simulink subsystem "CMS"  (R2024b)
settings: Solver=VariableStepAuto  StartTime=0.0  StopTime=10.0  RelTol=1e-3
undefined symbols (not defined in the file): Ts
settings Model: Creator=Kyle  LastModifiedBy=CD8435

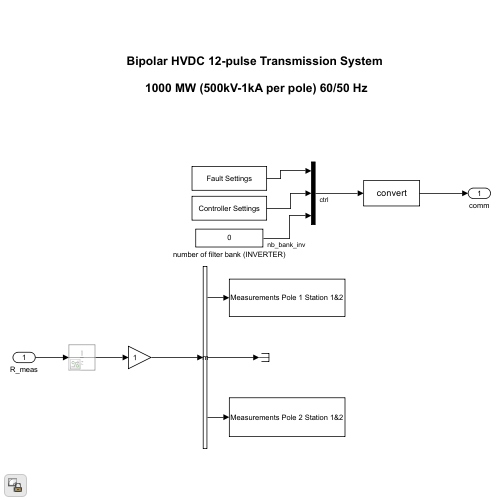
[thumbnail: Simulink's stored preview of the top-level diagram]
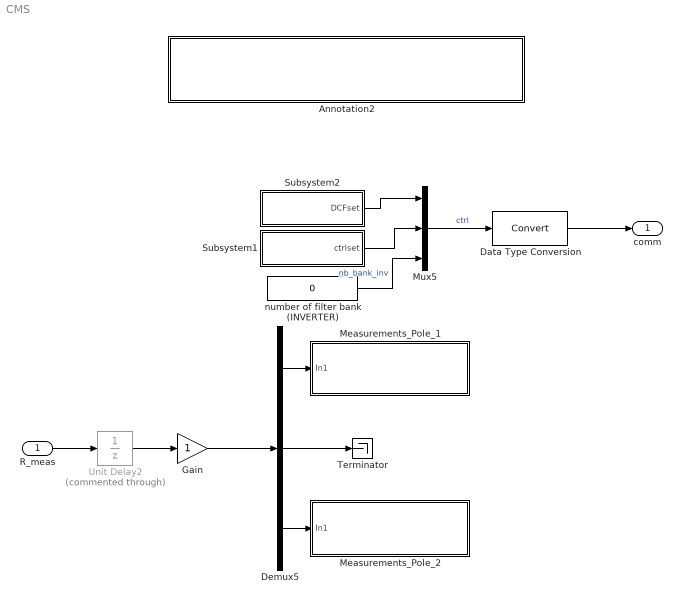
== system CMS ==
  R_meas : Inport
  Annotation2 : Subsystem  mask(Annotation){desc=|, maj=off, HZ=center, color=[0.9 0.9 0.9]}
      mask desc=|
      | Bipolar HVDC 12-pulse Transmission System
      | \n 1000 MW (500kV-1kA per pole) 60/50 Hz
      mask prompts: desc "Description (use \n for line return) :"; maj "Capital letters ?"; HZ "Horizontal Alignment"; color "Color [R G B] :"
      mask help: Annotation
      mask init:
      | if maj == 1 desc =upper(desc); end;
      | if strcmp(HZ, 'left') x = 0.05; end;
      | if strcmp(HZ, 'right') x = 0.95; end;
      | if strcmp(HZ, 'center') x = 0.50; end;
      mask TypeOptions HZ: left | right | center
      mask Display:
      | text(x, 0.50, desc, ...
      | 'horizontalAlignment', HZ, ...
      | 'verticalAlignment', 'middle') ;
  Data Type Conversion : DataTypeConversion  SaturateOnIntegerOverflow=off  RndMeth=Floor
  Demux5 : Demux  Outputs=[56 1 56]
      settings: DisplayOption=none
  Gain : Gain
  Measurements_Pole_1 : Subsystem
      mask Display: disp('Measurements Pole 1 Station 1&2')
  Measurements_Pole_2 : Subsystem
      mask Display: disp('Measurements Pole 2 Station 1&2')
  Mux5 : Mux  Inputs=3
  Subsystem1 : Subsystem
      mask Display: disp('Controller Settings')
  Subsystem2 : Subsystem
      mask Display: disp('Fault Settings')
  Terminator : Terminator
  Unit Delay2 : UnitDelay  Commented=through  SampleTime=Ts  HasFrameUpgradeWarning=on
  number of filter bank (INVERTER) : Constant  Value=0
  comm : Outport
  wires:
  Subsystem1/1(ctrlset) -> Mux5/2
  Subsystem2/1(DCFset) -> Mux5/1
  Mux5/1 -> Data Type Conversion/1  "ctrl"
  R_meas/1 -> Unit Delay2/1
  Demux5/1 -> Measurements_Pole_1/1(In1)
  Demux5/3 -> Measurements_Pole_2/1(In1)
  Demux5/2 -> Terminator/1
  Unit Delay2/1 -> Gain/1
  Gain/1 -> Demux5/1
  Data Type Conversion/1 -> comm/1
  number of filter bank (INVERTER)/1 -> Mux5/3  "nb_bank_inv"

== system CMS/Annotation2 ==
  note: Used only to display simulation parameters
  note: Text :
      | - justife a gauche
      | - Tahoma 10 Bold

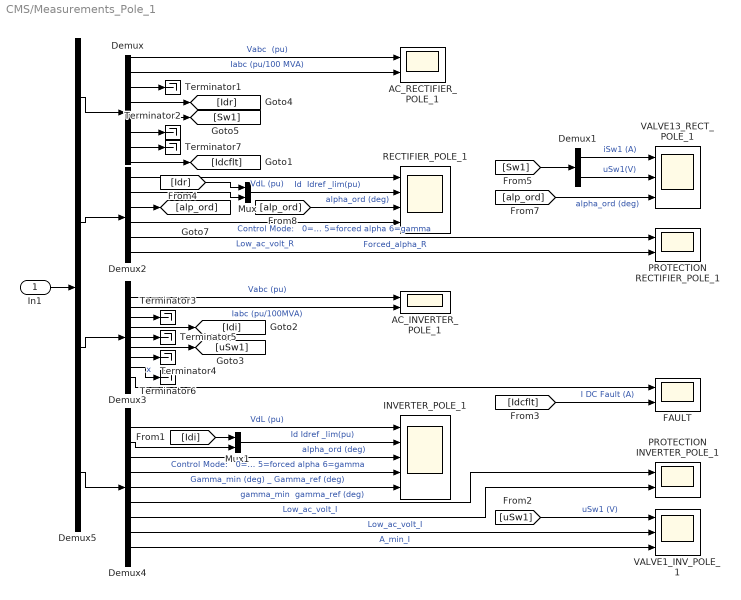
== system CMS/Measurements_Pole_1 ==
  In1 : Inport
  AC_INVERTER_POLE_1 : Scope  NumInputPorts=2
  AC_RECTIFIER_POLE_1 : Scope  NumInputPorts=2
  Demux : Demux  Outputs=[3 3 1 1 2 2 1 1]
  Demux1 : Demux  Outputs=[1 1]
      settings: DisplayOption=none
  Demux2 : Demux  Outputs=6
  Demux3 : Demux  Outputs="[3 3 1 1 12 1  1 1 1]"
  Demux4 : Demux  Outputs=[ 2 1 1 1 2 1 1 2 1]
  Demux5 : Demux  Outputs=[14 6 24 12]
      settings: DisplayOption=none
  FAULT : Scope  NumInputPorts=2
  INVERTER_POLE_1 : Scope  NumInputPorts=5
  Mux : Mux  Inputs=2
  Mux1 : Mux  Inputs=2
  PROTECTION INVERTER_POLE_1 : Scope  NumInputPorts=2
  PROTECTION RECTIFIER_POLE_1 : Scope  NumInputPorts=2
  RECTIFIER_POLE_1 : Scope  NumInputPorts=4
  Terminator{1..7} (7 alike) : Terminator
  VALVE13_RECT_POLE_1 : Scope  NumInputPorts=3
  VALVE1_INV_POLE_1 : Scope  NumInputPorts=3
  wires:
  In1/1 -> Demux5/1
  Demux/7 -> Terminator7/1
  Demux/8 -> [Idcflt]
  Demux3/8 -> Terminator6/1  "x"
  Demux3/9 -> FAULT/1
  [alp_ord] -> RECTIFIER_POLE_1/3  "alpha_ord (deg)"
  Demux2/3 -> [alp_ord]
  [alp_ord] -> VALVE13_RECT_POLE_1/3  "alpha_ord (deg)"
  [Sw1] -> Demux1/1
  [Idr] -> Mux/1
  [uSw1] -> VALVE1_INV_POLE_1/1  "uSw1 (V)"
  [Idi] -> Mux1/1
  [Idcflt] -> FAULT/2  "I DC Fault (A)"
  Demux3/7 -> Terminator4/1
  Demux5/4 -> Demux4/1
  Demux5/3 -> Demux3/1
  Demux5/2 -> Demux2/1
  Demux5/1 -> Demux/1
  Demux4/9 -> VALVE1_INV_POLE_1/3  "A_min_I"
  Demux4/7 -> PROTECTION INVERTER_POLE_1/2  "Low_ac_volt_I"
  Demux4/6 -> PROTECTION INVERTER_POLE_1/1  "gamma_min  gamma_ref (deg)"
  Demux3/5 -> Terminator5/1
  Demux3/3 -> Terminator3/1
  Demux3/6 -> [uSw1]
  Demux3/4 -> [Idi]
  Demux/6 -> Terminator2/1
  Demux/3 -> Terminator1/1
  Demux2/6 -> PROTECTION RECTIFIER_POLE_1/2  "Forced_alpha_R"
  Demux/4 -> [Idr]
  Demux/5 -> [Sw1]
  Demux4/8 -> VALVE1_INV_POLE_1/2  "Low_ac_volt_I"
  Demux1/2 -> VALVE13_RECT_POLE_1/2  "uSw1(V)"
  Demux1/1 -> VALVE13_RECT_POLE_1/1  "iSw1 (A)"
  Demux4/5 -> INVERTER_POLE_1/5  "Gamma_min (deg) _ Gamma_ref (deg)"
  Demux4/1 -> INVERTER_POLE_1/1  "VdL (pu)"
  Demux4/4 -> INVERTER_POLE_1/4  "Control Mode:   0=blked  1=curr 2=volt 3=alpha min  4=alpha max 5=forced alpha 6=gamma"
  Mux1/1 -> INVERTER_POLE_1/2  "Id Idref _lim(pu)"
  Demux4/2 -> Mux1/2
  Demux2/2 -> Mux/2
  Mux/1 -> RECTIFIER_POLE_1/2  "Id  Idref _lim(pu)"
  Demux2/5 -> PROTECTION RECTIFIER_POLE_1/1  "Low_ac_volt_R"
  Demux/1 -> AC_RECTIFIER_POLE_1/1  "Vabc  (pu)"
  Demux/2 -> AC_RECTIFIER_POLE_1/2  "Iabc (pu/100 MVA)"
  Demux2/1 -> RECTIFIER_POLE_1/1  "VdL (pu)"
  Demux3/1 -> AC_INVERTER_POLE_1/1  "Vabc (pu)"
  Demux3/2 -> AC_INVERTER_POLE_1/2  "Iabc (pu/100MVA)"
  Demux4/3 -> INVERTER_POLE_1/3  "alpha_ord (deg)"
  Demux2/4 -> RECTIFIER_POLE_1/4  "Control Mode:   0=blked  1=curr 2=volt 3=alpha min  4=alpha max 5=forced alpha 6=gamma"

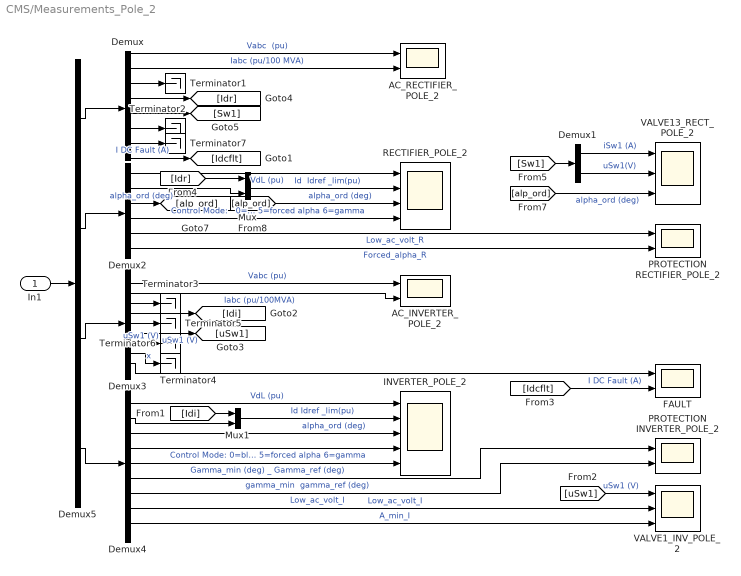
== system CMS/Measurements_Pole_2 ==
  In1 : Inport
  AC_INVERTER_POLE_2 : Scope  NumInputPorts=2
  AC_RECTIFIER_POLE_2 : Scope  NumInputPorts=2
  Demux : Demux  Outputs=[3 3 1 1 2 2 1 1]
  Demux1 : Demux  Outputs=[1 1]
      settings: DisplayOption=none
  Demux2 : Demux  Outputs=6
  Demux3 : Demux  Outputs="[3 3 1 1 12 1  1 1 1]"
  Demux4 : Demux  Outputs=[ 2 1 1 1 2 1 1 2 1]
  Demux5 : Demux  Outputs=[14 6 24 12]
      settings: DisplayOption=none
  FAULT : Scope  NumInputPorts=2
  INVERTER_POLE_2 : Scope  NumInputPorts=5
  Mux : Mux  Inputs=2
  Mux1 : Mux  Inputs=2
  PROTECTION INVERTER_POLE_2 : Scope  NumInputPorts=2
  PROTECTION RECTIFIER_POLE_2 : Scope  NumInputPorts=2
  RECTIFIER_POLE_2 : Scope  NumInputPorts=4
  Terminator{1..7} (7 alike) : Terminator
  VALVE13_RECT_POLE_2 : Scope  NumInputPorts=3
  VALVE1_INV_POLE_2 : Scope  NumInputPorts=3
  wires:
  Demux2/4 -> RECTIFIER_POLE_2/4  "Control Mode:   0=blked  1=curr 2=volt 3=alpha min  4=alpha max 5=forced alpha 6=gamma"
  Demux4/3 -> INVERTER_POLE_2/3  "alpha_ord (deg)"
  Demux3/2 -> AC_INVERTER_POLE_2/2  "Iabc (pu/100MVA)"
  Demux3/1 -> AC_INVERTER_POLE_2/1  "Vabc (pu)"
  Demux2/1 -> RECTIFIER_POLE_2/1  "VdL (pu)"
  Demux/2 -> AC_RECTIFIER_POLE_2/2  "Iabc (pu/100 MVA)"
  Demux/1 -> AC_RECTIFIER_POLE_2/1  "Vabc  (pu)"
  Demux2/5 -> PROTECTION RECTIFIER_POLE_2/1  "Low_ac_volt_R"
  Mux/1 -> RECTIFIER_POLE_2/2  "Id  Idref _lim(pu)"
  Demux2/2 -> Mux/2
  Demux4/2 -> Mux1/2
  Mux1/1 -> INVERTER_POLE_2/2  "Id Idref _lim(pu)"
  Demux4/4 -> INVERTER_POLE_2/4  "Control Mode: 0=blk 1=curr 2=volt 3=alpha min  4=alpha max 5=forced alpha 6=gamma"
  Demux4/1 -> INVERTER_POLE_2/1  "VdL (pu)"
  Demux4/5 -> INVERTER_POLE_2/5  "Gamma_min (deg) _ Gamma_ref (deg)"
  Demux1/1 -> VALVE13_RECT_POLE_2/1  "iSw1 (A)"
  Demux1/2 -> VALVE13_RECT_POLE_2/2  "uSw1(V)"
  Demux4/8 -> VALVE1_INV_POLE_2/2  "Low_ac_volt_I"
  Demux/5 -> [Sw1]
  Demux/4 -> [Idr]
  Demux2/6 -> PROTECTION RECTIFIER_POLE_2/2  "Forced_alpha_R"
  Demux/3 -> Terminator1/1
  Demux/6 -> Terminator2/1
  Demux3/4 -> [Idi]
  Demux3/6 -> [uSw1]  "uSw1 (V)"
  Demux3/3 -> Terminator3/1
  Demux3/5 -> Terminator5/1
  Demux4/6 -> PROTECTION INVERTER_POLE_2/1  "gamma_min  gamma_ref (deg)"
  Demux4/7 -> PROTECTION INVERTER_POLE_2/2  "Low_ac_volt_I"
  Demux4/9 -> VALVE1_INV_POLE_2/3  "A_min_I"
  Demux5/1 -> Demux/1
  Demux5/2 -> Demux2/1
  Demux5/3 -> Demux3/1
  Demux5/4 -> Demux4/1
  Demux3/7 -> Terminator6/1  "uSw1 (V)"
  [Idcflt] -> FAULT/2  "I DC Fault (A)"
  [Idi] -> Mux1/1
  [uSw1] -> VALVE1_INV_POLE_2/1  "uSw1 (V)"
  [Idr] -> Mux/1
  [Sw1] -> Demux1/1
  [alp_ord] -> VALVE13_RECT_POLE_2/3  "alpha_ord (deg)"
  Demux2/3 -> [alp_ord]  "alpha_ord (deg)"
  [alp_ord] -> RECTIFIER_POLE_2/3  "alpha_ord (deg)"
  Demux3/9 -> FAULT/1
  Demux3/8 -> Terminator4/1  "x"
  Demux/8 -> [Idcflt]
  Demux/7 -> Terminator7/1  "I DC Fault (A)"
  In1/1 -> Demux5/1

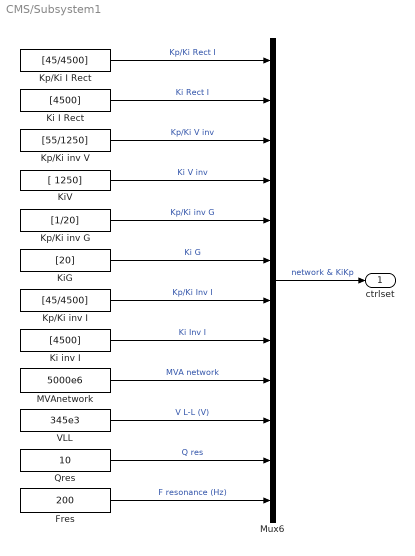
== system CMS/Subsystem1 ==
  " KiV" : Constant  Value=[ 1250]
  Fres : Constant  Value=200
  Ki I Rect : Constant  Value=[4500]
  Ki inv I : Constant  Value=[4500]
  KiG : Constant  Value=[20]
  Kp/Ki I Rect : Constant  Value=[45/4500]
  Kp/Ki inv G : Constant  Value=[1/20]
  Kp/Ki inv I : Constant  Value=[45/4500]
  Kp/Ki inv V : Constant  Value=[55/1250]
  MVAnetwork : Constant  Value=5000e6
  Mux6 : Mux  Inputs=[1 1 1 1 1 1 1 1 1 1 1 1]
  Qres : Constant  Value=10
  VLL : Constant  Value=345e3
  ctrlset : Outport
  wires:
  Qres/1 -> Mux6/11  "Q res"
  Ki inv I/1 -> Mux6/8  "Ki Inv I"
  Kp/Ki inv I/1 -> Mux6/7  "Kp/Ki Inv I"
  KiG/1 -> Mux6/6  "Ki G"
  VLL/1 -> Mux6/10  "V L-L (V)"
  Fres/1 -> Mux6/12  "F resonance (Hz)"
  MVAnetwork/1 -> Mux6/9  "MVA network"
  Mux6/1 -> ctrlset/1  "network & KiKp"
  Kp/Ki inv G/1 -> Mux6/5  "Kp/Ki inv G"
  " KiV"/1 -> Mux6/4  "Ki V inv"
  Kp/Ki inv V/1 -> Mux6/3  "Kp/Ki V inv"
  Ki I Rect/1 -> Mux6/2  "Ki Rect I"
  Kp/Ki I Rect/1 -> Mux6/1  "Kp/Ki Rect I"

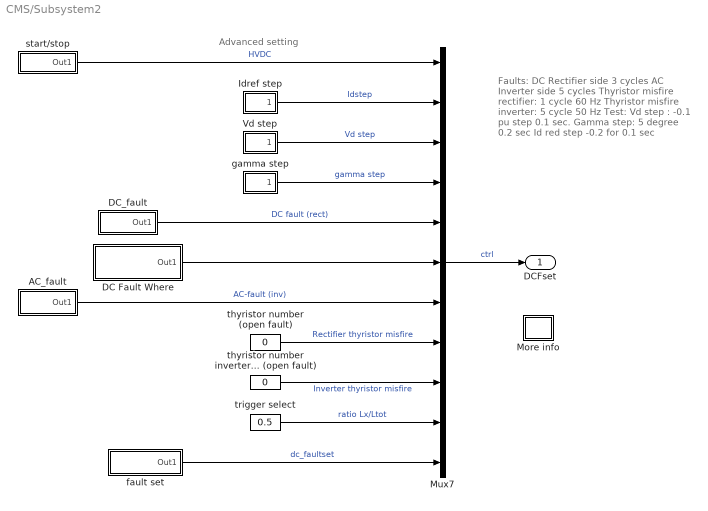
== system CMS/Subsystem2 ==
  note: Faults:
      | DC Rectifier side 3 cycles
      | AC Inverter side 5 cycles
      | Thyristor misfire rectifier: 1 cycle 60 Hz
      | Thyristor misfire inverter: 5 cycle 50 Hz
      |
      | Test:
      | Vd step  : -0.1 pu step 0.1 sec.
      | Gamma step: 5 degree 0.2 sec
      | Id red step -0.2 for 0.1 sec
  note: Advanced setting
  AC_fault : Subsystem  mask(fault_type){fault=0:no fault}
      mask prompts: fault "fault type"
      mask help:
      | fault_tpye:
      | 0:no fault
      | 1:phase-a fault
      | 2:phase-ab fault
      | 3:phase-abc fault
      mask init:
      | if fault==1
      | 	x='no fault';
      | elseif fault==2
      | 	x='a fault';
      | elseif fault==3
      | 	x='ab fault';	
      | else
      | 	x='abc fault';
      | end
      mask TypeOptions fault: 0:no fault | 1:phase-a fault  | 2:phase-ab fault  | 3:phase-abc fault
      mask Display: disp(x)
  DC Fault Where : Subsystem  mask{DC_fault_where=Pole 1 Only}
      mask prompts: DC_fault_where "DC Fault on which pole?"
      mask init:
      | if DC_fault_where == 1
      | 	x = 'Both Poles';
      | elseif DC_fault_where == 2
      | 	x = 'Pole 1 Only';
      | elseif DC_fault_where == 3
      | 	x = 'Pole 2 Only';
      | end
      mask TypeOptions DC_fault_where: Both Poles | Pole 1 Only | Pole 2 Only
      mask Display: disp(x)
  DC_fault : Subsystem  mask{on=off}
      mask init:
      | if on==1
      | 	x='on';
      | else
      | 	x='off';
      | end
      mask Display: disp(x)
  Idref step : Subsystem  mask{on=off}
      mask init:
      | if on==1
      | 	x='on';
      | else
      | 	x='off';
      | end
      mask Display: disp(x)
  More info : Subsystem
      mask Display: disp('?')
  Mux7 : Mux  Inputs=11
  Vd step : Subsystem  mask{on=off}
      mask init:
      | if on==1
      | 	x='on';
      | else
      | 	x='off';
      | end
      mask Display: disp(x)
  fault set : Subsystem  mask(fault set){Tacq=0.5, Tst=[0.05 0 10], Tdr=[0.01 0 10]}
      mask prompts: Tacq "acquisition period"; Tst "fault start time set [Tst, Tst_var, Tst_pd]"; Tdr "fault duration set [Tst, Tst_var, Tst_pd]"
      mask help:
      | output dimention: 7=1+3+3
      |
      | acquisition period, Tacq
      |
      | fault start time set [Tst, Tst_var, Tst_pd]
      | if Tst_var=0, fault starts at Tst
      | if Tst_var<>0, Tst varies from Tst to Tst+Tst_var, variation cycle is Tst_pd.
      |
      | fault duration set [Tdr, Tdr_var, Tdr_pd]
      | if Tdr_var=0, fault durstion is fixed, equal Tdr
      | if Tdr_var<>0, fault duration varies from Tdr to Tdr+Tdr_var, variation cycle is Tdr_pd.
      mask Display: disp(Tacq)
  gamma step : Subsystem  mask{on=off}
      mask init:
      | if on==1
      | 	x='on';
      | else
      | 	x='off';
      | end
      mask Display: disp(x)
  start/stop : Subsystem  mask{on=on}
      mask init:
      | if on==1
      | 	x='on';
      | else
      | 	x='off';
      | end
      mask Display: disp(x)
  thyristor number (open fault) : Constant  Value=0
  thyristor number inverter (open fault) : Constant  Value=0
  trigger select : Constant  Value=0.5
  DCFset : Outport
  wires:
  fault set/1(Out1) -> Mux7/11  "dc_faultset"
  DC Fault Where/1(Out1) -> Mux7/6
  start/stop/1(Out1) -> Mux7/1  "HVDC"
  Mux7/1 -> DCFset/1  "ctrl"
  trigger select/1 -> Mux7/10  "ratio Lx/Ltot"
  thyristor number inverter (open fault)/1 -> Mux7/9  "Inverter thyristor misfire"
  thyristor number (open fault)/1 -> Mux7/8  "Rectifier thyristor misfire"
  AC_fault/1(Out1) -> Mux7/7  "AC-fault (inv)"
  DC_fault/1(Out1) -> Mux7/5  "DC fault (rect)"
  gamma step/1(Out1) -> Mux7/4  "gamma step"
  Vd step/1(Out1) -> Mux7/3  "Vd step"
  Idref step/1(Out1) -> Mux7/2  "Idstep"

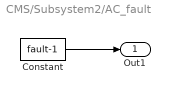
== system CMS/Subsystem2/AC_fault ==
  Constant : Constant  Value=fault-1
  Out1 : Outport  InitialOutput=0
  wires:
  Constant/1 -> Out1/1

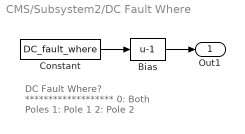
== system CMS/Subsystem2/DC Fault Where ==
  note: DC Fault Where?
      | *******************
      | 0: Both Poles
      | 1: Pole 1
      | 2: Pole 2
  Bias : Bias  Bias=-1  SaturateOnIntegerOverflow=off
  Constant : Constant  Value=DC_fault_where
  Out1 : Outport  InitialOutput=0
  wires:
  Constant/1 -> Bias/1
  Bias/1 -> Out1/1

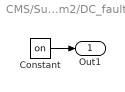
== system CMS/Subsystem2/DC_fault ==
  Constant : Constant  Value=on
  Out1 : Outport  InitialOutput=0
  wires:
  Constant/1 -> Out1/1

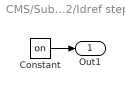
== system CMS/Subsystem2/Idref step ==
  Constant : Constant  Value=on
  Out1 : Outport  InitialOutput=0
  wires:
  Constant/1 -> Out1/1

== system CMS/Subsystem2/More info ==
  note: In the DC Fault block, change the multiplication factor of 1 in the Switching times to 100, so that the DC fault is now eliminated. In the A-G Fault block, change to 1 the 100 multiplication factor in the
      | Switching times so that a 6 cycles  line-to-ground fault is now applied at t = 0.7 s. The Low AC voltage detection (LACVD) subsystem in the rectifier and inverter protections and the Commutation
      | Failure Prevention Control (CFPREV) in the inverter protection are activated by default. Restart the simulation.
      |
      | Notice the 120 Hz oscillations in the DC voltage and currents during the fault. When the fault is cleared at t = 0.8 s,  the VDCOL operates and reduces the reference current to 0.3 pu. The system
      | recovers in approximately 0.35 s after fault clearing.  The  LACVD detects the fault and locks the DC Fault  protection  that should not detect a DC fault even if the DC line voltage dips.  Look at the
      | CFPREV output (A_min_I) which decreases the maximum delay angle limit in order to increase the commutation margin during and after the fault. Now deactivate the CFPREV protection by
      | deselecting  the "ON State" in the CFPREV dilaog box. Restart the simulation and observe the difference in  recovery time of the DC transmission. Note that a  commutation failure now occurs during
      | the recovery.  A commutation failure is the result of a failure of the incoming valve to take over the direct current before the commutation voltage reverses its polarity.  The symptoms are  a zero DC
      | voltage accros the affected bridge  causing an increase of the DC current at a rate determined mainly by the DC circuit inductance.
  note: AC line-to-ground fault at the inverter
  note: Deactivate the steps applied on the current reference and on the voltage reference in the Master Control and in the inverter control respectively by setting the switches in lower position. In the DC
      | Fault block, change to 1 the 100 multiplication factor in the Switching times so that a fault is now applied at t = 0.7 s. Reduce the Simulation stop time from 2 to 1.4 s. The DC Fault protection (DCPROT)
      | in the rectifier is activated by default. Open the FAULT scope to observe the DC fault current. Restart the simulation.
      |
      | At fault application the DC current quickly increases to 2.3 pu and the DC voltage falls to zero at the rectifier. This DC voltages drop is seen by the Voltage Dependant Currrent Order Limiter (VDCOL)
      | which reduces the reference current to 0.3 pu at the rectifier. A DC current still continues to circulate in the fault. Then, at t = 0.77 s, the rectifier alpha firing angle is forced to 166 degrees by the DC
      | protection because  a DC voltage drop is detected (VdL< 0.5 pu for more than 70 ms). The rectifier now operates in inverter mode. The DC line voltage becomes negative and the energy stored in the
      | line is returned to the AC network, causing rapid extinction of the fault current at its next zero-crossing. Then, alpha is released at t = 0.87 s and the normal DC voltage and current recover in
      | approximately 0.4 s.
  note: DC line fault at the rectifier
  note: Start-up and Stop
  note: DEMONSTRATION
  note: A 1000 MW (500 kV, 2kA) DC linterconnexion is used to transmit power from a 500 kV, 5000 MVA, 60 Hz network to a  345 kV, 10 000 MVA, 50 Hz network.
      |
      | The rectifier and the inverter are 12-pulse converters using two 6-pulse thyristor bridges connected in series. The rectifier and the inverter are interconnected through a 300 km distributed
      | parameter line and two 0.5 H smoothing reactors. The transformer tap changers are not simulated and  fixed taps are assumed. Open the two transformer blocks in the Rectifier and Inverter
      | subsystems to see the factors applied on the primary voltage: 0.90 on rectifier side and 0.96 on inverter side. Reactive power required by the converters is provided by a set of capacitor banks
      | plus 11th, 13th and  high pass filters for a total of  600 Mvar on each side. Two circuit breakers are used to apply faults on the inverter AC side and rectifier DC side.
      |
      | The rectifier and inverter control systems use the  Discrete 12-pulse HVDC Control block of the Extras/Discrete Control Blocks library. DC Protection functions are implemented in each converter.
      | At the rectifier the DC fault protection will detect and force the delay angle into the inverter region so to extinguish the fault current. At the inverter the commutation failure prevention control will
      | detect AC faults and reduce the maximum delay angle limit in order to decrease the risk of commutation failure. The Low AC voltage detection blocks will lock the DC fault protection when a drop in
      | the AC voltage is detected. The Master Control block initiates the starting and stopping of the converters as well as the ramping up and down of the current references. The power system and the
      | control system are both  discretized for a sample time Ts=50 us. Notice that the "Model initialization" function of the model  automatically sets Ts = 50e-6 in your Matlab workspace. A description of
      | the control systems is provided in the HVDC Transmission System Case Study of the User's Manual.
  note: Steady-state and transient performance of a 12-pulse,
      | 1000 MW (500 kV-2kA) 50/60 Hz HVDC transmission system
  note: CIRCUIT DESCRIPTION
  note: The system is programmed to start and  reach a steady state. Then steps are applied on the reference current of the rectifier and  on the inverter reference voltage in order to observe the dynamic
      | response  of the regulators. Finally, a stop sequence is initiated to bring the DC power down before blocking the converters. Start the simulation. Open the RECTIFIER and INVERTER scopes (in the
      | Data Acquisition subsystem) and observe the DC line voltage  on trace 1 (1pu = 500 kV) and the DC line current  (reference and mesured values)  on trace 2 (1pu = 2kA).
  note: Verify in the Master Control that the "Enable Ref. Current Step"  switch is in the upper position. This switch is used to apply a step on the reference voltage. Also verify that the  reference voltage
      | step is enabled in the Inverter Control. At t=0.7 s, a -0.2 pu step is first applied on the reference current (decrease from 1 pu  to 0.8 pu ) and at t=0.8 s,  the reference current is reset to its 1 pu
      | original value.The current stabilizes in  approximately 0.1 seconds. Steps are also  applied on the reference voltage of the inverter (-0.1 pu / +0.1 pu at t=1.0 s / 1.1s. )
  note: Step response of curent and voltage regulators
  note: Silvano Casoria (Hydro-Quebec)
  note: In the Master Control, the converters are deblocked and started by ramping the rectifier and inverter reference current. At t = 0.02 s (i.e. when the converters at deblocked), the reference current
      | is ramped to reach the minimum value of 0.1 pu in 0.3 s (0.33 pu/s). At the end of this first ramp (t = 0.32 s) the DC line is charged at its nominal voltage and DC voltage reaches steady-state. At
      | t= 0.4 s,  the reference current is ramped from 0.1 pu to 1 pu (2kA) in 0.18 s (5 pu/s). At the end of this starting sequence (t=0.58 s) , the DC current reaches steady state. The RECTIFIER then
      | controls the current and the INVERTER controls the voltage. In steady-state, the alpha firing angles (trace 3) are 16.5 degrees and 143 degrees respectively on the RECTIFIER and INVERTER sides.
      | The exctinction angle gamma (minimum value) is measured at the INVERTER  and shown in trace 4. In steady-state, the minimum value is between 22 and 24 degrees. The control mode of operation
      | (an  integer between 0 to 6) is shown in trace 4 (0= blocked; 1=Current control; 2=Voltage control; 3=Alpha minimum limitation;  4=Alpha maximum limitation; 5=Forced or constant alpha;
      | 6=Gamma control). At t = 1.4 s the Stop sequence is initiated by ramping down the current to 0.1 pu. At t = 1.6 s a Forced-alpha at the Rectifier extinguishes the current and at the Inverter the
      | Forced-alpha brings down the DC voltage. At t = 1.7 s the pulses are blocked in both converters.

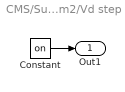
== system CMS/Subsystem2/Vd step ==
  Constant : Constant  Value=on
  Out1 : Outport  InitialOutput=0
  wires:
  Constant/1 -> Out1/1

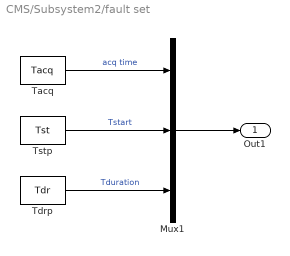
== system CMS/Subsystem2/fault set ==
  Mux1 : Mux  Inputs="[1 3 3  ]"
  Tacq : Constant  Value=Tacq
  Tdrp : Constant  Value=Tdr
  Tstp : Constant  Value=Tst
  Out1 : Outport  InitialOutput=0
  wires:
  Mux1/1 -> Out1/1
  Tdrp/1 -> Mux1/3  "Tduration"
  Tstp/1 -> Mux1/2  "Tstart"
  Tacq/1 -> Mux1/1  "acq time"

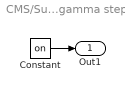
== system CMS/Subsystem2/gamma step ==
  Constant : Constant  Value=on
  Out1 : Outport  InitialOutput=0
  wires:
  Constant/1 -> Out1/1

== system CMS/Subsystem2/start//stop ==
  Constant : Constant  Value=on
  Out1 : Outport  InitialOutput=0
  wires:
  Constant/1 -> Out1/1
